simulink library "rotations_lib"  (R2023b)
settings: Solver=VariableStepAuto  StartTime=0.0  StopTime=10.0  RelTol=1e-3
settings Model: Creator=Nabil  LastModifiedBy=luke
settings DebuggingCC: UnconnectedInputMsg=warning  UnconnectedOutputMsg=warning  UnconnectedLineMsg=warning
settings ModelReferenceCC: EnableRefExpFcnMdlSchedulingChecks=on
settings RTWCC: DLArmComputeVersion=19.05

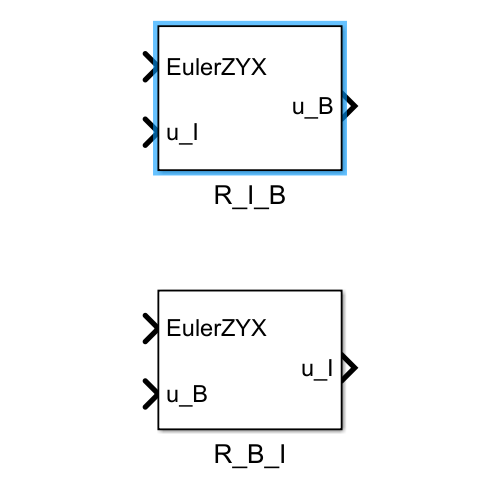
[thumbnail: Simulink's stored preview of the top-level diagram]
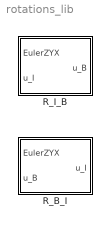
== system rotations_lib ==
  R_B_I : Subsystem
  R_I_B : Subsystem

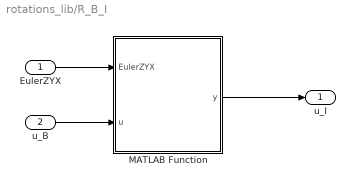
== system rotations_lib/R_B_I ==
  EulerZYX : Inport
  u_B : Inport  Port=2  PortDimensions=3
  MATLAB Function : MATLAB Function  TreatAsAtomicUnit=on
  u_I : Outport
  wires:
  EulerZYX/1 -> MATLAB Function/1(EulerZYX)
  MATLAB Function/1(y) -> u_I/1
  u_B/1 -> MATLAB Function/2(u)

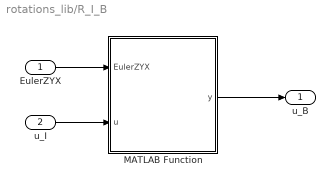
== system rotations_lib/R_I_B ==
  EulerZYX : Inport
  u_I : Inport  Port=2  PortDimensions=3
  MATLAB Function : MATLAB Function  TreatAsAtomicUnit=on
  u_B : Outport
  wires:
  MATLAB Function/1(y) -> u_B/1
  u_I/1 -> MATLAB Function/2(u)
  EulerZYX/1 -> MATLAB Function/1(EulerZYX)

== matlab function rotations_lib/R_I_B/MATLAB Function ==
  data: EulerZYX input; u input; y output
function y = R_I_B(EulerZYX, u)
%This function creates a rotation matrix to rotate the vector U from the
%inertial frame to the body frame. this rotation matrix is Tait-Bryan ZYX
%intrinsic, active rotation.

%Creating euler angle inputs
psi = EulerZYX(1); %yaw about Z
theta = EulerZYX(2); %pitch about y
phi   = EulerZYX(3); %roll about x

%Create rotation matrix from intertial frame to body frame
R_ib= rotz(psi)*roty(theta)*rotx(phi);

%y is the body vector obtained by rotating the inertial vector u by
%rotation matrix R_ib
y = R_ib*u;

end

== matlab function rotations_lib/R_B_I/MATLAB Function ==
  data: EulerZYX input; u input; y output
function y = R_B_I(EulerZYX, u)
%This function creates a rotation matrix to rotate the vector U from the
%body frame to the inertial frame. this rotation matrix is Tait-Bryan ZYX
%intrinsic, active rotation.

%Creating euler angle inputs
psi = EulerZYX(1); %yaw about Z
theta = EulerZYX(2); %pitch about y
phi   = EulerZYX(3); %roll about x

%Create rotation matrix from intertial frame to body frame
R_ib= rotz(psi)*roty(theta)*rotx(phi);

%transpose rotation matrix to get the inverse, R_bi
R_bi = R_ib.';

%y is the intertial vector obtained by rotating the body vector u by
%rotation matrix R_bi
y = R_bi*u;

end
